simulink library "ChimeControlLibBtc"  (R2022b)
settings: Solver=VariableStepAuto  StartTime=0.0  StopTime=10.0  RelTol=1e-3
undefined symbols (not defined in the file or in its folder): chime_group_count, Row, spkrRouting
libraries: dspindex x10, RTC x3, FeaturePath x2, TOP x2, TuneVar x2, HandyTextFile x1
(part 1 of 2)
settings Model: Creator=kl13806  LastModifiedBy=kl13806
settings SolverCC: AlgebraicLoopSolver=TrustRegion
settings DebuggingCC: UnconnectedInputMsg=warning  UnconnectedOutputMsg=warning  UnconnectedLineMsg=warning  SFMachineParentedDataDiag=warning
settings ModelReferenceCC: EnableRefExpFcnMdlSchedulingChecks=on
settings RTWCC: DLArmComputeVersion=19.05

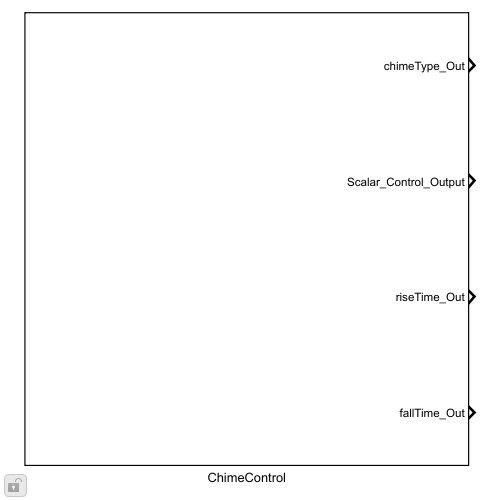
[thumbnail: Simulink's stored preview of the top-level diagram]
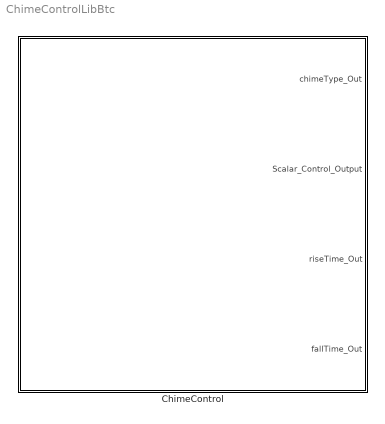
== system ChimeControlLibBtc ==
  ChimeControl : Subsystem  mask(Chimes ChimeControl){Config=[], FeatureName=Control}
      mask prompts: Config "ChimeControlConfig"; FeatureName "Feature path name:"
      mask init:
      | blkh=gcbh;
      | Config=BTConfig.Assert(blkh,Config);
      | 
      | Config.Validate();
      | BTConfig.InitSetFeatureIfPresent(blkh,'FeatureName');
      | 
      | % Flatten variables used by MFBs:
      | %nch=Config.Nch;
      mask Callback Config: BTConfig.CallbackHideIfPresent(gcbh,{'FeatureName'});
      mask TypeOptions FeatureName: FeaturePath/FeatureName

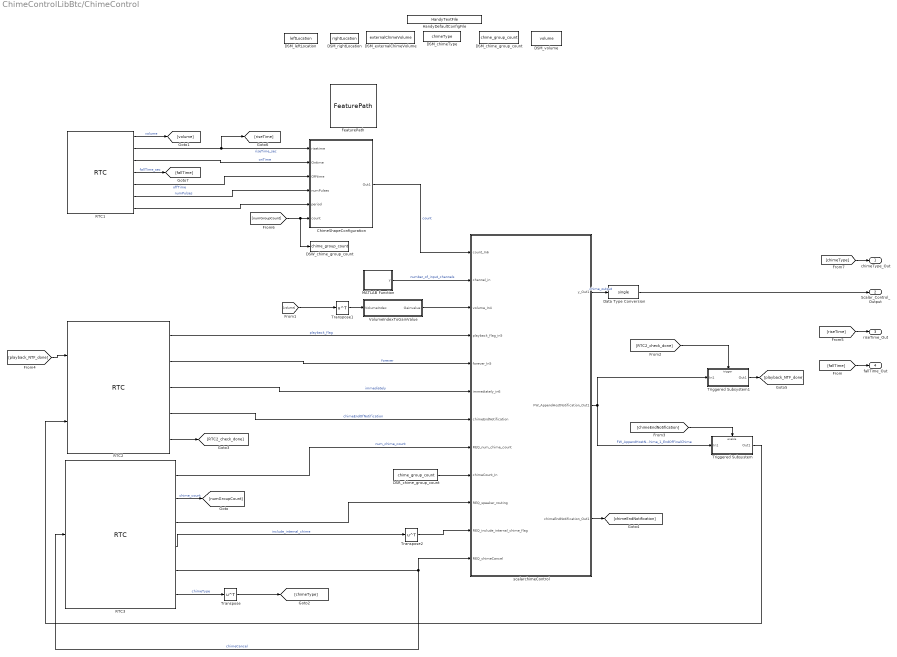
== system ChimeControlLibBtc/ChimeControl ==
  ChimeShapeConfiguration : Subsystem
  DSM_chimeType : DataStoreMemory  DataStoreName=chimeType  ShowAdditionalParam=off
  DSM_chime_group_count : DataStoreMemory  DataStoreName=chime_group_count  InitialValue=ones(1, Config.Nch)  ShowAdditionalParam=off
  DSM_externalChimeVolume : DataStoreMemory  DataStoreName=externalChimeVolume  InitialValue=zeros(1,Config.Nch)  ShowAdditionalParam=off
  DSM_leftLocation : DataStoreMemory  DataStoreName=leftLocation  ShowAdditionalParam=off
  DSM_rightLocation : DataStoreMemory  DataStoreName=rightLocation  ShowAdditionalParam=off
  DSM_volume : DataStoreMemory  DataStoreName=volume  InitialValue=Config.Volume  ShowAdditionalParam=off
  DSR_chime_group_count : DataStoreRead  DataStoreName=chime_group_count  IndexOptions=Index vector (dialog)  Indices=1  OutputSizes=1
  DSW_chime_group_count : DataStoreWrite  DataStoreName=chime_group_count  IndexOptions=Index vector (dialog)  Indices=1  OutputSizes=1
  Data Type Conversion : DataTypeConversion  OutDataTypeStr=single  SaturateOnIntegerOverflow=off  RndMeth=Floor
  FeaturePath : FeaturePath/FeaturePath  FeatureName=Control  IsGroup=off  GroupNumber=-1  IsModule=off  TriggerInit=[800 149 915 256]
  HandyDefaultConfigFile : HandyTextFile/HandyTextFile  TemplateSource=Config  FileSuffix=Init  OpenDialogOnLoad=off  UseThisBlockName=off  TheDefaultText=|  ShowInLibBrowser=on
      | % $(FILENAME) Setup model parameters for each "Init" callback (e.g. update diagram)
      | sample_rate_in_hertz = 44100;
      | frame_size = 32;
      | sysin_channel_count = 2;
  MATLAB Function : MATLAB Function  TreatAsAtomicUnit=on
  RTC1 : RTC/RTC  REQ_Priority=RTC_Mask.NormalPriority  RequestAtInit=off  EnableRequest=off  REQElemName1=volume  REQElemType1=single  REQElemWidth1=length(Config.Volume)  REQElemInitial1=Config.Volume  REQElemName2=riseTime  REQElemType2=single  REQElemWidth2=length(Config.RiseTime)  REQElemInitial2=Config.RiseTime  REQElemName3=onTime  REQElemType3=single  REQElemWidth3=length(Config.OnTime)  REQElemInitial3=Config.OnTime  REQElemName4=fallTime  REQElemType4=single  REQElemWidth4=length(Config.FallTime)  REQElemInitial4=Config.FallTime  REQElemName5=offTime  REQElemType5=single  REQElemWidth5=length(Config.OffTime)  REQElemInitial5=Config.OffTime  REQElemName6=numPulses  REQElemType6=int32  REQElemWidth6=length(Config.NumPulses)  REQElemInitial6=Config.NumPulses  REQElemName7=period  REQElemType7=single  REQElemWidth7=length(Config.Period)  REQElemInitial7=Config.Period  REQElemType8=uint32  REQElemWidth8=1  REQElemInitial8=[]  REQElemType9=uint32  REQElemWidth9=1  REQElemInitial9=[]  REQElemType10=uint32  REQElemWidth10=1  REQElemInitial10=[]  EnableResponse=on  EnableRSP_StatusIn=off  RSPElemType1=uint32  RSPElemWidth1=1  RSPElemType2=uint32  RSPElemWidth2=1  RSPElemType3=uint32  RSPElemWidth3=1  RSPElemType4=uint32  RSPElemWidth4=1  RSPElemType5=uint32  RSPElemWidth5=1  RSPElemType6=uint32  RSPElemWidth6=1  RSPElemType7=uint32  RSPElemWidth7=1  RSPElemType8=uint32  RSPElemWidth8=1  RSPElemType9=uint32  RSPElemWidth9=1  RSPElemType10=uint32  RSPElemWidth10=1  EnableNotification=off  EnableNTF_PrepTrig=off  NTFElemType1=uint32  NTFElemWidth1=1  NTFElemType2=uint32  NTFElemWidth2=1  NTFElemType3=uint32  NTFElemWidth3=1  NTFElemType4=uint32  NTFElemWidth4=1  NTFElemType5=uint32  NTFElemWidth5=1  NTFElemType6=uint32  NTFElemWidth6=1  NTFElemType7=uint32  NTFElemWidth7=1  NTFElemType8=uint32  NTFElemWidth8=1  NTFElemType9=uint32  NTFElemWidth9=1  NTFElemType10=uint32  NTFElemWidth10=1  MaskMessageName=PulseConfig
  RTC2 : RTC/RTC  REQ_Priority=RTC_Mask.NormalPriority  RequestAtInit=off  EnableRequest=off  REQElemName1=PlaybackSignal  REQElemType1=int32  REQElemWidth1=length(Config.PlaybackFlag)  REQElemInitial1=Config.PlaybackFlag  REQElemName2=Forever  REQElemType2=boolean  REQElemWidth2=length(Config.Forever)  REQElemInitial2=Config.Forever  REQElemName3=Immediately  REQElemType3=boolean  REQElemWidth3=length(Config.Immediately)  REQElemInitial3=Config.Immediately  REQElemName4=ChimeEndNotification  REQElemType4=boolean  REQElemWidth4=length(Config.ChimeEndNotification)  REQElemInitial4=Config.ChimeEndNotification  REQElemType5=uint32  REQElemWidth5=1  REQElemInitial5=[]  REQElemType6=uint32  REQElemWidth6=1  REQElemInitial6=[]  REQElemType7=uint32  REQElemWidth7=1  REQElemInitial7=[]  REQElemType8=uint32  REQElemWidth8=1  REQElemInitial8=[]  REQElemType9=uint32  REQElemWidth9=1  REQElemInitial9=[]  REQElemType10=uint32  REQElemWidth10=1  REQElemInitial10=[]  EnableResponse=on  EnableRSP_StatusIn=off  RSPElemType1=uint32  RSPElemWidth1=1  RSPElemType2=uint32  RSPElemWidth2=1  RSPElemType3=uint32  RSPElemWidth3=1  RSPElemType4=uint32  RSPElemWidth4=1  RSPElemType5=uint32  RSPElemWidth5=1  RSPElemType6=uint32  RSPElemWidth6=1  RSPElemType7=uint32  RSPElemWidth7=1  RSPElemType8=uint32  RSPElemWidth8=1  RSPElemType9=uint32  RSPElemWidth9=1  RSPElemType10=uint32  RSPElemWidth10=1  EnableNotification=on  EnableNTF_PrepTrig=off  NTFElemName1=FW_AppendHostNotification  NTFElemType1=boolean  NTFElemWidth1=length(Config.ChimeEndNotification)  NTFElemType2=uint32  NTFElemWidth2=1  NTFElemType3=uint32  NTFElemWidth3=1  NTFElemType4=uint32  NTFElemWidth4=1  NTFElemType5=uint32  NTFElemWidth5=1  NTFElemType6=uint32  NTFElemWidth6=1  NTFElemType7=uint32  NTFElemWidth7=1  NTFElemType8=uint32  NTFElemWidth8=1  NTFElemType9=uint32  NTFElemWidth9=1  NTFElemType10=uint32  NTFElemWidth10=1  MaskMessageName=StatePlayback
  RTC3 : RTC/RTC  REQ_Priority=RTC_Mask.NormalPriority  RequestAtInit=off  EnableRequest=off  REQElemName1=NumChimeCount  REQElemType1=int32  REQElemWidth1=length(Config.NumChimeCount)  REQElemInitial1=Config.NumChimeCount  REQElemName2=NumGroupCount  REQElemType2=int32  REQElemWidth2=length(chime_group_count)  REQElemInitial2=chime_group_count  REQElemName3=SpeakerRouting  REQElemType3=int32  REQElemWidth3=length(spkrRouting)  REQElemInitial3=spkrRouting  REQElemName4=IncludeInternalChimeFlag  REQElemType4=boolean  REQElemWidth4=length(Config.IncludeInternalChimeFlag)  REQElemInitial4=Config.IncludeInternalChimeFlag  REQElemName5=ChimeCancel  REQElemType5=boolean  REQElemWidth5=length(Config.ChimeCancel)  REQElemInitial5=Config.ChimeCancel  REQElemName6=ChimeType  REQElemType6=single  REQElemWidth6=length(Config.ChimeType)  REQElemInitial6=Config.ChimeType  REQElemType7=boolean  REQElemWidth7=1  REQElemInitial7=[]  REQElemType8=int32  REQElemWidth8=1  REQElemInitial8=[]  REQElemType9=int32  REQElemWidth9=1  REQElemInitial9=[]  REQElemType10=int32  REQElemWidth10=1  REQElemInitial10=[]  EnableResponse=on  EnableRSP_StatusIn=off  RSPElemName1=chimeCancelAck  RSPElemType1=boolean  RSPElemWidth1=length(Config.ChimeCancel)  RSPElemType2=uint32  RSPElemWidth2=1  RSPElemType3=uint32  RSPElemWidth3=1  RSPElemType4=uint32  RSPElemWidth4=1  RSPElemType5=uint32  RSPElemWidth5=1  RSPElemType6=uint32  RSPElemWidth6=1  RSPElemType7=uint32  RSPElemWidth7=1  RSPElemType8=uint32  RSPElemWidth8=1  RSPElemType9=uint32  RSPElemWidth9=1  RSPElemType10=uint32  RSPElemWidth10=1  EnableNotification=off  EnableNTF_PrepTrig=off  NTFElemType1=uint32  NTFElemWidth1=1  NTFElemType2=uint32  NTFElemWidth2=1  NTFElemType3=uint32  NTFElemWidth3=1  NTFElemType4=uint32  NTFElemWidth4=1  NTFElemType5=uint32  NTFElemWidth5=1  NTFElemType6=uint32  NTFElemWidth6=1  NTFElemType7=uint32  NTFElemWidth7=1  NTFElemType8=uint32  NTFElemWidth8=1  NTFElemType9=uint32  NTFElemWidth9=1  NTFElemType10=uint32  NTFElemWidth10=1  MaskMessageName=ChimesFeature
  Transpose : Math  Operator=transpose  SignedPower=on
  Transpose1 : Math  Operator=transpose  SignedPower=on
  Transpose2 : Math  Operator=transpose  SignedPower=on
  Triggered Subsystem : Subsystem  TreatAsAtomicUnit=on
  Triggered Subsystem1 : Subsystem  TreatAsAtomicUnit=on
  VolumeIndexToGainValue : Subsystem
  scalarchimeControl : Subsystem
  chimeType_Out : Outport  VectorParamsAs1DForOutWhenUnconnected=off
  Scalar_Control_Output : Outport  Port=2  VectorParamsAs1DForOutWhenUnconnected=off
  riseTime_Out : Outport  Port=3  VectorParamsAs1DForOutWhenUnconnected=off
  fallTime_Out : Outport  Port=4  VectorParamsAs1DForOutWhenUnconnected=off
  wires:
  Data Type Conversion/1 -> Scalar_Control_Output/1
  VolumeIndexToGainValue/1(Gainvalue) -> scalarchimeControl/3(volume_In4)
  RTC1/2 -> ChimeShapeConfiguration/1(risetime), [riseTime]  "riseTime_sec"
  RTC2/3 -> scalarchimeControl/6(immediately_in6)  "immediately"
  RTC3/5 -> scalarchimeControl/12(REQ_chimeCancel), RTC3/1  "chimeCancel"
  scalarchimeControl/1(y_Out1) -> Data Type Conversion/1  "chime_output"
  RTC2/1 -> scalarchimeControl/4(playback_flag_in5)  "playback_flag"
  Transpose2/1 -> scalarchimeControl/11(REQ_include_internal_chime_flag)
  RTC1/3 -> ChimeShapeConfiguration/2(Ontime)  "onTime"
  DSR_chime_group_count/1 -> scalarchimeControl/9(chimeCount_In)
  RTC3/1 -> scalarchimeControl/8(REQ_num_chime_count)  "num_chime_count"
  RTC2/4 -> scalarchimeControl/7(chimeEndNotification)  "chimeEndOfNotification"
  ChimeShapeConfiguration/1(Out1) -> scalarchimeControl/1(count_In6)  "count"
  RTC2/2 -> scalarchimeControl/5(forever_In5)  "forever"
  Transpose1/1 -> VolumeIndexToGainValue/1(VolumeIndex)
  Triggered Subsystem/1(Out1) -> RTC2/2
  RTC1/5 -> ChimeShapeConfiguration/3(Offtime)  "offTime"
  RTC3/6 -> Transpose/1  "chimeType"
  scalarchimeControl/2(FW_AppendHostNotification_Out1) -> Triggered Subsystem/1(In1), Triggered Subsystem1/1(In1)  "FW_AppendHostNotification_0_StartOfFinalChime_1_EndOfFinalChime"
  RTC3/4 -> Transpose2/1  "include_internal_chime"
  RTC3/3 -> scalarchimeControl/10(REQ_speaker_routing)
  RTC1/7 -> ChimeShapeConfiguration/5(period)
  RTC1/1 -> [volume]  "volume"
  [volume] -> Transpose1/1
  Transpose/1 -> [chimeType]
  RTC2/5 -> [RTC2_check_done]
  [RTC2_check_done] -> Triggered Subsystem1/Trigger
  scalarchimeControl/3(chimeEndNotification_Out1) -> [chimeEndNotification]
  [chimeEndNotification] -> Triggered Subsystem/Enable
  Triggered Subsystem1/1(Out1) -> [playback_NTF_done]
  [playback_NTF_done] -> RTC2/1
  RTC1/6 -> ChimeShapeConfiguration/4(numPulses)  "numPulses"
  RTC1/4 -> [fallTime]  "fallTime_sec"
  [riseTime] -> riseTime_Out/1
  [fallTime] -> fallTime_Out/1
  RTC3/2 -> [numGroupCount]  "chime_count"
  [numGroupCount] -> DSW_chime_group_count/1, ChimeShapeConfiguration/6(count)
  [chimeType] -> chimeType_Out/1
  MATLAB Function/1(y) -> scalarchimeControl/2(channel_in)  "number_of_input_channels"

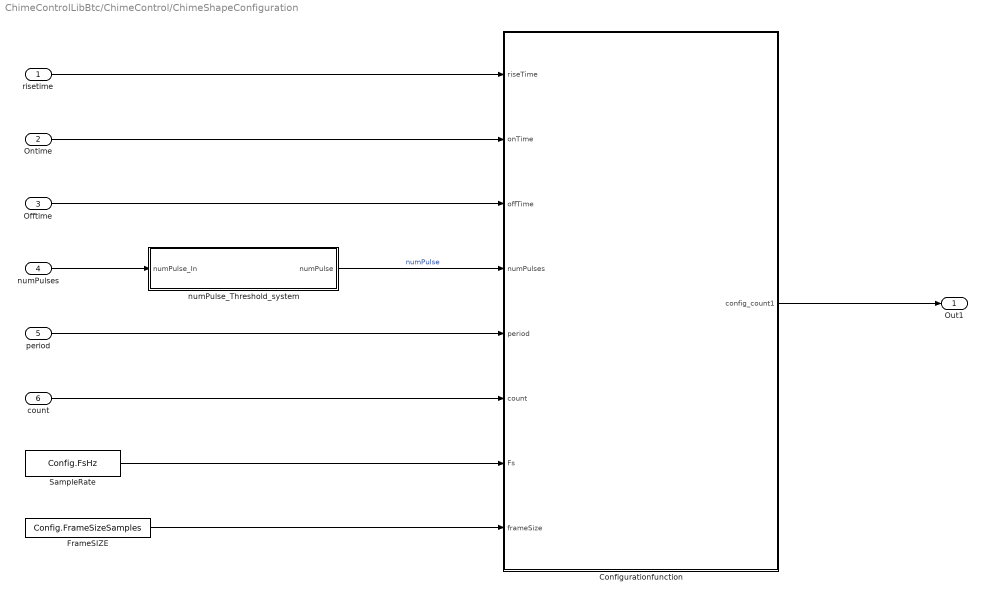
== system ChimeControlLibBtc/ChimeControl/ChimeShapeConfiguration ==
  risetime : Inport
  Ontime : Inport  Port=2
  Offtime : Inport  Port=3
  numPulses : Inport  Port=4
  period : Inport  Port=5
  count : Inport  Port=6
  Configurationfunction : MATLAB Function  TreatAsAtomicUnit=on
  FrameSIZE : Constant  Value=Config.FrameSizeSamples  OutDataTypeStr=single
  SampleRate : Constant  Value=Config.FsHz  OutDataTypeStr=single
  numPulse_Threshold_system : Subsystem
  Out1 : Outport  VectorParamsAs1DForOutWhenUnconnected=off
  wires:
  FrameSIZE/1 -> Configurationfunction/8(frameSize)
  SampleRate/1 -> Configurationfunction/7(Fs)
  count/1 -> Configurationfunction/6(count)
  Offtime/1 -> Configurationfunction/3(offTime)
  Configurationfunction/1(config_count1) -> Out1/1
  period/1 -> Configurationfunction/5(period)
  Ontime/1 -> Configurationfunction/2(onTime)
  risetime/1 -> Configurationfunction/1(riseTime)
  numPulses/1 -> numPulse_Threshold_system/1(numPulse_In)
  numPulse_Threshold_system/1(numPulse) -> Configurationfunction/4(numPulses)  "numPulse"

== system ChimeControlLibBtc/ChimeControl/Triggered Subsystem ==
  In1 : Inport
  Enable : EnablePort
  Data Type Conversion : DataTypeConversion  OutDataTypeStr=int32  SaturateOnIntegerOverflow=off  RndMeth=Floor
  Out1 : Outport  VectorParamsAs1DForOutWhenUnconnected=off
  wires:
  In1/1 -> Data Type Conversion/1
  Data Type Conversion/1 -> Out1/1

== system ChimeControlLibBtc/ChimeControl/Triggered Subsystem1 ==
  In1 : Inport
  Trigger : TriggerPort  TriggerType=function-call  VariantControl=Variant
  Constant : Constant
  Equal : RelationalOperator  Operator===  OutDataTypeStr=boolean  RndMeth=Simplest  InputSameDT=off
  Variable Selector : dspindex/Variable Selector  NumInputs=1  rowsOrCols=Columns  IdxMode=Fixed  Elements=[1]  ZerOneIdxMode=One-based  errmode=Clip Index  FillMode=on  FillValues=0
  Out1 : Outport  VectorParamsAs1DForOutWhenUnconnected=off
  wires:
  Variable Selector/1 -> Out1/1
  Constant/1 -> Equal/2
  Equal/1 -> Variable Selector/1
  In1/1 -> Equal/1

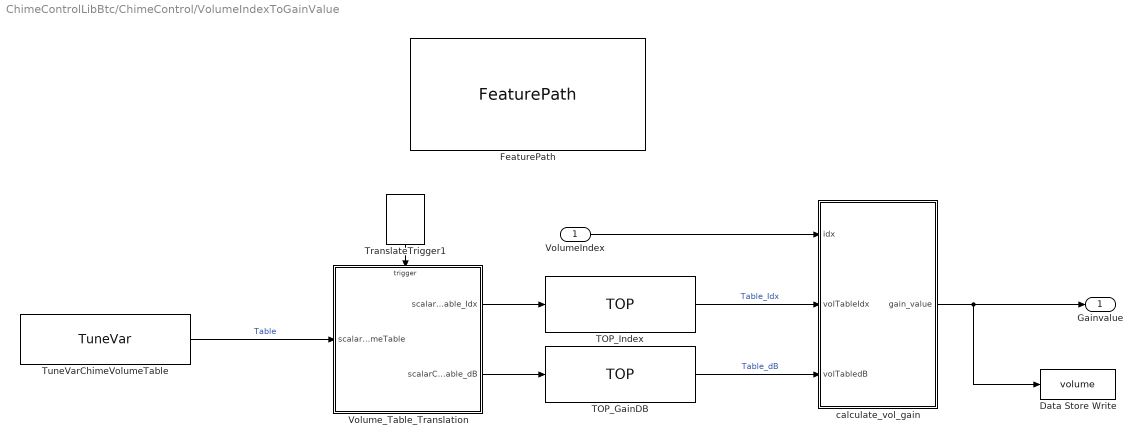
== system ChimeControlLibBtc/ChimeControl/VolumeIndexToGainValue ==
  VolumeIndex : Inport
  Data Store Write : DataStoreWrite  DataStoreName=volume  IndexOptions=Index vector (dialog)  Indices=1  OutputSizes=1
  FeaturePath : FeaturePath/FeaturePath  FeatureName=chimeVolume  IsGroup=off  GroupNumber=-1  IsModule=off  TriggerInit=[360 -1 595 111]
  TOP_GainDB : TOP/TOP  TriggerInit=[495 307 645 363]  TopName=Table_dB  DataType=Inherit: Same as input  BankNumber=0  PreOverlay=false  PostOverlay=false  Role=Automatic
  TOP_Index : TOP/TOP  TriggerInit=[495 237 645 293]  TopName=Table_Idx  DataType=Inherit: Same as input  BankNumber=0  PreOverlay=false  PostOverlay=false  Role=Automatic
  TranslateTrigger1 : TuneVar/TranslateTrigger  TriggerInit=[336 155 374 205]
  TuneVarChimeVolumeTable : TuneVar/TuneVar  Description=|  TuneName=Table  SpecifyMaxSize=off  VariableDim=1 (Row)  MaxSize=[2 11]  TunabilityNumber=2  MinValue=[0;-100]  MaxValue=[1;0]  TriggerInit=[-30 275 140 325]  MaskValue=[[1 32 64 96 128 160 192 224 230 240 250] / 255; [-126.5 -100 -90 -40 -30 -20 -10 0.0 6.0206 10 20]]
      | <HTML>Gain table maps index to gain.
      | The index values are <FONT color="red">normalized</Font> floats between 0 and 1 while the gains are in dB (i.e. 0 implies no attenuation).
      | </html>
  Volume_Table_Translation : MATLAB Function  TreatAsAtomicUnit=on
  calculate_vol_gain : MATLAB Function  TreatAsAtomicUnit=on
  Gainvalue : Outport  VectorParamsAs1DForOutWhenUnconnected=off
  wires:
  TOP_GainDB/1 -> calculate_vol_gain/3(volTabledB)  "Table_dB"
  Volume_Table_Translation/2(scalarChimeControl_Table_dB) -> TOP_GainDB/1
  TuneVarChimeVolumeTable/1 -> Volume_Table_Translation/1(scalarChimeControl_VolumeTable)  "Table"
  Volume_Table_Translation/1(scalarChimeControl_Table_Idx) -> TOP_Index/1
  TOP_Index/1 -> calculate_vol_gain/2(volTableIdx)  "Table_Idx"
  calculate_vol_gain/1(gain_value) -> Data Store Write/1, Gainvalue/1
  TranslateTrigger1/1 -> Volume_Table_Translation/Trigger
  VolumeIndex/1 -> calculate_vol_gain/1(idx)

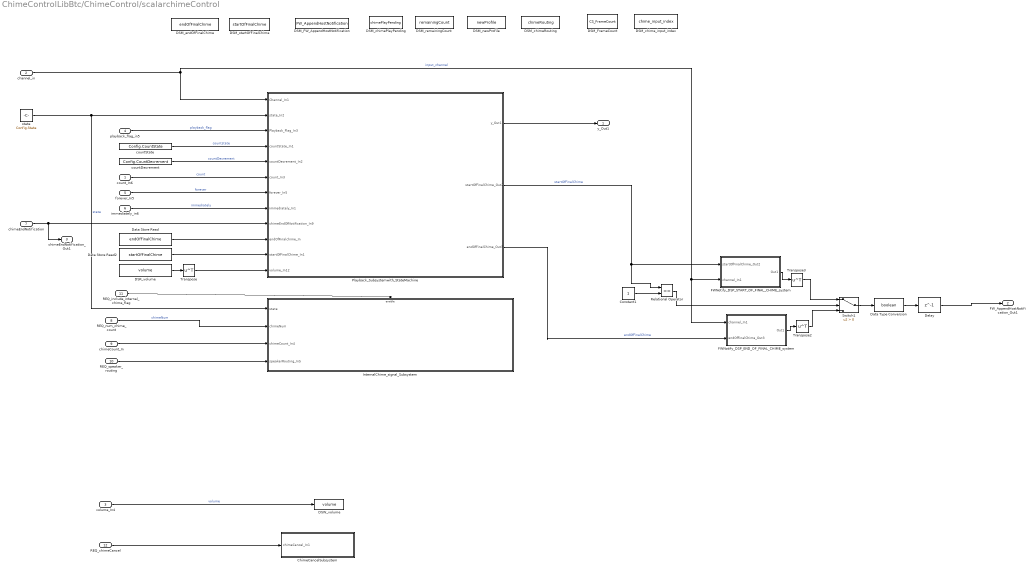
== system ChimeControlLibBtc/ChimeControl/scalarchimeControl ==
  count_In6 : Inport
  channel_in : Inport  Port=2
  volume_In4 : Inport  Port=3
  playback_flag_in5 : Inport  Port=4
  forever_In5 : Inport  Port=5
  immediately_in6 : Inport  Port=6
  chimeEndNotification : Inport  Port=7
  REQ_num_chime_count : Inport  Port=8
  chimeCount_In : Inport  Port=9
  REQ_speaker_routing : Inport  Port=10
  REQ_include_internal_chime_flag : Inport  Port=11
  REQ_chimeCancel : Inport  Port=12
  ChimeCancelSubsystem : Subsystem
  Constant1 : Constant  OutDataTypeStr=single
  DSM_FW_AppendHostNotification : DataStoreMemory  DataStoreName=FW_AppendHostNotification  InitialValue=zeros(1,Config.Nch)  ShowAdditionalParam=off
  DSM_FrameCount : DataStoreMemory  DataStoreName=CS_FrameCount  ShowAdditionalParam=off  OutDataTypeStr=int32
  DSM_chimePlayPending : DataStoreMemory  DataStoreName=chimePlayPending  InitialValue=zeros(1,Config.Nch)  ShowAdditionalParam=off  OutDataTypeStr=int32
  DSM_chimeRouting : DataStoreMemory  DataStoreName=chimeRouting  InitialValue=zeros(1,Config.Nch)  ShowAdditionalParam=off  OutDataTypeStr=int32
  DSM_chime_input_index : DataStoreMemory  DataStoreName=chime_input_index  InitialValue=Config.ChimeInputIndex  ShowAdditionalParam=off
  DSM_endOfFinalChime : DataStoreMemory  DataStoreName=endOfFinalChime  InitialValue=zeros(1,Config.Nch)  VectorParams1D=off  ShowAdditionalParam=off  OutDataTypeStr=boolean
  DSM_newProfile : DataStoreMemory  DataStoreName=newProfile  ShowAdditionalParam=off  OutDataTypeStr=int32
  DSM_remainingCount : DataStoreMemory  DataStoreName=remainingCount  ShowAdditionalParam=off  OutDataTypeStr=int32
  DSM_startOfFinalChime : DataStoreMemory  DataStoreName=startOfFinalChime  InitialValue=zeros(1,Config.Nch)  VectorParams1D=off  ShowAdditionalParam=off  OutDataTypeStr=boolean
  DSR_volume : DataStoreRead  DataStoreName=volume  IndexOptions=Index vector (dialog)  Indices=1  OutputSizes=1
  DSW_volume : DataStoreWrite  DataStoreName=volume  IndexOptions=Index vector (dialog)  Indices=1  OutputSizes=1
  Data Store Read : DataStoreRead  DataStoreName=endOfFinalChime  IndexOptions=Index vector (dialog)  Indices=1  OutputSizes=1
  Data Store Read2 : DataStoreRead  DataStoreName=startOfFinalChime  IndexOptions=Index vector (dialog)  Indices=1  OutputSizes=1
  Data Type Conversion : DataTypeConversion  OutDataTypeStr=boolean  SaturateOnIntegerOverflow=off  RndMeth=Floor
  Delay : Delay  DelayLength=1  InputProcessing=Columns as channels (frame based)
  FWNotify_DSP_END_OF_FINAL_CHIME_system : Subsystem  TreatAsAtomicUnit=on
  FWNotify_DSP_START_OF_FINAL_CHIME_system : Subsystem  TreatAsAtomicUnit=on
  InternalChime_signal_Subsystem : Subsystem
  Playback_Subsystemwith_StateMachine : Subsystem
  Relational Operator : RelationalOperator  Operator===  OutDataTypeStr=boolean  RndMeth=Simplest  InputSameDT=off
  Switch1 : Switch  Criteria=u2 > Threshold  SaturateOnIntegerOverflow=off  InputSameDT=off
  Transpose : Math  Operator=transpose  SignedPower=on
  Transpose2 : Math  Operator=transpose  SignedPower=on
  Transpose3 : Math  Operator=transpose  SignedPower=on
  countDecrement : Constant  Value=Config.CountDecrement  VectorParams1D=off  OutDataTypeStr=single
  countState : Constant  Value=Config.CountState  VectorParams1D=off  OutDataTypeStr=single
  state : Constant  Value=Config.State  VectorParams1D=off  OutDataTypeStr=single
  y_Out1 : Outport  VectorParamsAs1DForOutWhenUnconnected=off
  FW_AppendHostNotification_Out1 : Outport  Port=2  VectorParamsAs1DForOutWhenUnconnected=off
  chimeEndNotification_Out1 : Outport  Port=3  VectorParamsAs1DForOutWhenUnconnected=off
  wires:
  Constant1/1 -> Relational Operator/2
  Data Store Read2/1 -> Playback_Subsystemwith_StateMachine/11(startOfFinalChime_In1)
  Transpose/1 -> Playback_Subsystemwith_StateMachine/12(volume_In12)
  DSR_volume/1 -> Transpose/1
  volume_In4/1 -> DSW_volume/1  "volume"
  Data Store Read/1 -> Playback_Subsystemwith_StateMachine/10(endOfFinalchime_In)
  REQ_speaker_routing/1 -> InternalChime_signal_Subsystem/4(speakerRouting_In5)
  chimeCount_In/1 -> InternalChime_signal_Subsystem/3(chimeCount_In4)
  Playback_Subsystemwith_StateMachine/2(startOfFinalChime_Out2) -> Relational Operator/1, FWNotify_DSP_START_OF_FINAL_CHIME_system/1(startOfFinalChime_Out2)  "startOfFinalChime"
  Playback_Subsystemwith_StateMachine/3(endOfFinalChime_Out3) -> FWNotify_DSP_END_OF_FINAL_CHIME_system/2(endOfFinalChime_Out3)  "endOfFinalChime"
  chimeEndNotification/1 -> chimeEndNotification_Out1/1, Playback_Subsystemwith_StateMachine/9(chimeEndOfNotification_In9)
  countState/1 -> Playback_Subsystemwith_StateMachine/4(countState_In1)  "countstate"
  immediately_in6/1 -> Playback_Subsystemwith_StateMachine/8(immediately_In1)  "immediately"
  forever_In5/1 -> Playback_Subsystemwith_StateMachine/7(forever_In5)  "forever"
  count_In6/1 -> Playback_Subsystemwith_StateMachine/6(count_In3)  "count"
  countDecrement/1 -> Playback_Subsystemwith_StateMachine/5(countDecrement_In2)  "countDecrement"
  playback_flag_in5/1 -> Playback_Subsystemwith_StateMachine/3(Playback_Flag_In3)  "playback_flag"
  state/1 -> Playback_Subsystemwith_StateMachine/2(state_In2), InternalChime_signal_Subsystem/1(state)  "state"
  Playback_Subsystemwith_StateMachine/1(y_Out1) -> y_Out1/1
  REQ_include_internal_chime_flag/1 -> InternalChime_signal_Subsystem/Enable
  REQ_num_chime_count/1 -> InternalChime_signal_Subsystem/2(chimeNum)  "chimeNum"
  REQ_chimeCancel/1 -> ChimeCancelSubsystem/1(chimeCancel_In1)
  FWNotify_DSP_START_OF_FINAL_CHIME_system/1(Out1) -> Transpose3/1
  Transpose3/1 -> Switch1/1
  Delay/1 -> FW_AppendHostNotification_Out1/1
  channel_in/1 -> FWNotify_DSP_END_OF_FINAL_CHIME_system/1(channel_In1), FWNotify_DSP_START_OF_FINAL_CHIME_system/2(channel_In1), Playback_Subsystemwith_StateMachine/1(Channel_In1)  "input_channel"
  Switch1/1 -> Data Type Conversion/1
  FWNotify_DSP_END_OF_FINAL_CHIME_system/1(Out1) -> Transpose2/1
  Transpose2/1 -> Switch1/3
  Data Type Conversion/1 -> Delay/1
  Relational Operator/1 -> Switch1/2

== system ChimeControlLibBtc/ChimeControl/ChimeShapeConfiguration/numPulse_Threshold_system ==
  numPulse_In : Inport
  If Action Subsystem : Subsystem  TreatAsAtomicUnit=on
  If Action Subsystem1 : Subsystem  TreatAsAtomicUnit=on
  Relational Operator : RelationalOperator  OutDataTypeStr=boolean  RndMeth=Simplest  InputSameDT=off
  Switch : Switch  Criteria=u2 ~= 0  SaturateOnIntegerOverflow=off  InputSameDT=off
  thresholdNumPulse : Constant  Value=Config.ThresholdNumPulse  VectorParams1D=off  OutDataTypeStr=single
  numPulse : Outport  VectorParamsAs1DForOutWhenUnconnected=off
  wires:
  If Action Subsystem1/1(Out1) -> Switch/3
  If Action Subsystem/1(Out1) -> Switch/1
  Relational Operator/1 -> Switch/2
  Switch/1 -> numPulse/1  "numPulse"
  numPulse_In/1 -> If Action Subsystem/1(In1), Relational Operator/1
  thresholdNumPulse/1 -> If Action Subsystem1/1(In1), Relational Operator/2

== system ChimeControlLibBtc/ChimeControl/scalarchimeControl/ChimeCancelSubsystem ==
  chimeCancel_In1 : Inport
  If : If  IfExpression=u1 == 1
  If Action Subsystem : Subsystem  TreatAsAtomicUnit=on
  If Action Subsystem1 : Subsystem  TreatAsAtomicUnit=on
  wires:
  chimeCancel_In1/1 -> If/1
  If/1 -> If Action Subsystem/Action
  If/2 -> If Action Subsystem1/Action

== system ChimeControlLibBtc/ChimeControl/scalarchimeControl/FWNotify_DSP_END_OF_FINAL_CHIME_system ==
  channel_In1 : Inport
  endOfFinalChime_Out3 : Inport  Port=2
  Assignment : Assignment  DiagnosticForDimensions=Warning  IndexOptions=Index vector (port)  Indices=1  OutputSizes=1
  Assignment1 : Assignment  DiagnosticForDimensions=Warning  IndexOptions=Index vector (port)  Indices=1  OutputSizes=1
  Constant : Constant  VectorParams1D=off  OutDataTypeStr=single
  DSR_FW_AppendHostNotification : DataStoreRead  DataStoreName=FW_AppendHostNotification  IndexOptions=Index vector (dialog)  Indices=1  OutputSizes=1
  DSW_endOfFinalChime : DataStoreWrite  DataStoreName=endOfFinalChime  IndexOptions=Index vector (dialog)  Indices=1  OutputSizes=1
  Data Type Conversion : DataTypeConversion  OutDataTypeStr=boolean  SaturateOnIntegerOverflow=off  RndMeth=Floor
  Out1 : Outport  VectorParamsAs1DForOutWhenUnconnected=off
  wires:
  channel_In1/1 -> Assignment1/3, Assignment/3
  DSR_FW_AppendHostNotification/1 -> Assignment/1
  Constant/1 -> Data Type Conversion/1, Assignment/2
  Assignment/1 -> Out1/1
  Data Type Conversion/1 -> Assignment1/2
  Assignment1/1 -> DSW_endOfFinalChime/1
  endOfFinalChime_Out3/1 -> Assignment1/1

== system ChimeControlLibBtc/ChimeControl/scalarchimeControl/FWNotify_DSP_START_OF_FINAL_CHIME_system ==
  startOfFinalChime_Out2 : Inport
  channel_In1 : Inport  Port=2
  Assignment : Assignment  DiagnosticForDimensions=Warning  IndexOptions=Index vector (port)  Indices=1  OutputSizes=1
  Assignment1 : Assignment  DiagnosticForDimensions=Warning  IndexOptions=Index vector (port)  Indices=1  OutputSizes=1
  Constant : Constant  Value=0  OutDataTypeStr=single
  DSR_FW_AppendHostNotification : DataStoreRead  DataStoreName=FW_AppendHostNotification  IndexOptions=Index vector (dialog)  Indices=1  OutputSizes=1
  Data Store Write : DataStoreWrite  DataStoreName=startOfFinalChime  IndexOptions=Index vector (dialog)  Indices=1  OutputSizes=1
  Data Type Conversion : DataTypeConversion  OutDataTypeStr=boolean  SaturateOnIntegerOverflow=off  RndMeth=Floor
  Out1 : Outport  VectorParamsAs1DForOutWhenUnconnected=off
  wires:
  channel_In1/1 -> Assignment1/3, Assignment/3
  DSR_FW_AppendHostNotification/1 -> Assignment/1
  Constant/1 -> Data Type Conversion/1, Assignment/2
  Assignment/1 -> Out1/1
  Data Type Conversion/1 -> Assignment1/2
  Assignment1/1 -> Data Store Write/1
  startOfFinalChime_Out2/1 -> Assignment1/1

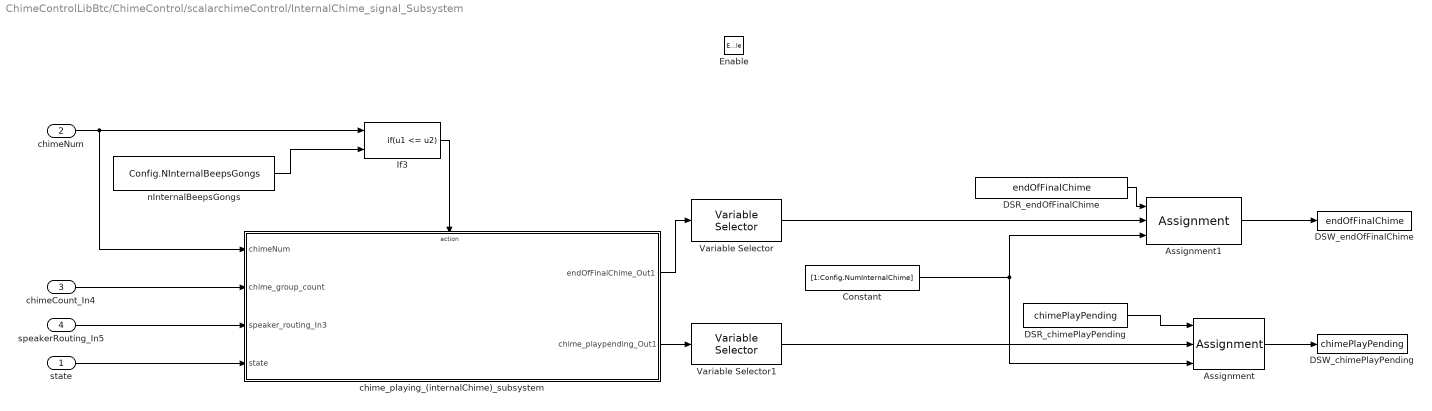
== system ChimeControlLibBtc/ChimeControl/scalarchimeControl/InternalChime_signal_Subsystem ==
  state : Inport
  chimeNum : Inport  Port=2
  chimeCount_In4 : Inport  Port=3
  speakerRouting_In5 : Inport  Port=4
  Enable : EnablePort
  Assignment : Assignment  DiagnosticForDimensions=Warning  IndexOptions=Index vector (port)  Indices=1  OutputSizes=1
  Assignment1 : Assignment  DiagnosticForDimensions=Warning  IndexOptions=Index vector (port)  Indices=1  OutputSizes=1
  Constant : Constant  Value=[1:Config.NumInternalChime]  OutDataTypeStr=single
  DSR_chimePlayPending : DataStoreRead  DataStoreName=chimePlayPending  IndexOptions=Index vector (dialog)  Indices=1  OutputSizes=1
  DSR_endOfFinalChime : DataStoreRead  DataStoreName=endOfFinalChime  IndexOptions=Index vector (dialog)  Indices=1  OutputSizes=1
  DSW_chimePlayPending : DataStoreWrite  DataStoreName=chimePlayPending  IndexOptions=Index vector (dialog)  Indices=1  OutputSizes=1
  DSW_endOfFinalChime : DataStoreWrite  DataStoreName=endOfFinalChime  IndexOptions=Index vector (dialog)  Indices=1  OutputSizes=1
  If3 : If  NumInputs=2  IfExpression=u1 <= u2  ShowElse=off
  Variable Selector : dspindex/Variable Selector  NumInputs=1  rowsOrCols=Columns  IdxMode=Fixed  Elements=[1:Config.NumInternalChime]  ZerOneIdxMode=One-based  errmode=Clip Index  FillMode=on  FillValues=0
  Variable Selector1 : dspindex/Variable Selector  NumInputs=1  rowsOrCols=Columns  IdxMode=Fixed  Elements=[1:Config.NumInternalChime]  ZerOneIdxMode=One-based  errmode=Clip Index  FillMode=on  FillValues=0
  chime_playing_(internalChime)_subsystem : Subsystem
  nInternalBeepsGongs : Constant  Value=Config.NInternalBeepsGongs  OutDataTypeStr=int32
  wires:
  If3/1 -> chime_playing_(internalChime)_subsystem/Action
  chimeCount_In4/1 -> chime_playing_(internalChime)_subsystem/2(chime_group_count)
  state/1 -> chime_playing_(internalChime)_subsystem/4(state)
  nInternalBeepsGongs/1 -> If3/2
  speakerRouting_In5/1 -> chime_playing_(internalChime)_subsystem/3(speaker_routing_In3)
  chimeNum/1 -> chime_playing_(internalChime)_subsystem/1(chimeNum), If3/1
  chime_playing_(internalChime)_subsystem/1(endOfFinalChime_Out1) -> Variable Selector/1
  chime_playing_(internalChime)_subsystem/2(chime_playpending_Out1) -> Variable Selector1/1
  Variable Selector/1 -> Assignment1/2
  Assignment1/1 -> DSW_endOfFinalChime/1
  Assignment/1 -> DSW_chimePlayPending/1
  DSR_chimePlayPending/1 -> Assignment/1
  Variable Selector1/1 -> Assignment/2
  DSR_endOfFinalChime/1 -> Assignment1/1
  Constant/1 -> Assignment/3, Assignment1/3

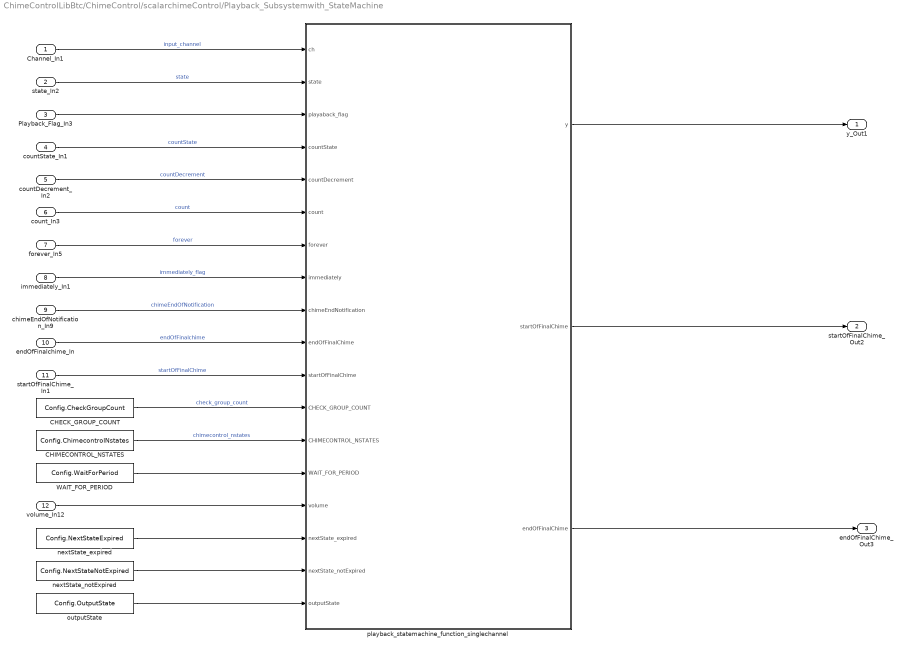
== system ChimeControlLibBtc/ChimeControl/scalarchimeControl/Playback_Subsystemwith_StateMachine ==
  Channel_In1 : Inport
  state_In2 : Inport  Port=2
  Playback_Flag_In3 : Inport  Port=3
  countState_In1 : Inport  Port=4
  countDecrement_In2 : Inport  Port=5
  count_In3 : Inport  Port=6
  forever_In5 : Inport  Port=7
  immediately_In1 : Inport  Port=8
  chimeEndOfNotification_In9 : Inport  Port=9
  endOfFinalchime_In : Inport  Port=10
  startOfFinalChime_In1 : Inport  Port=11
  volume_In12 : Inport  Port=12
  CHECK_GROUP_COUNT : Constant  Value=Config.CheckGroupCount  VectorParams1D=off  OutDataTypeStr=single
  CHIMECONTROL_NSTATES : Constant  Value=Config.ChimecontrolNstates  VectorParams1D=off  OutDataTypeStr=single
  WAIT_FOR_PERIOD : Constant  Value=Config.WaitForPeriod  VectorParams1D=off  OutDataTypeStr=single
  nextState_expired : Constant  Value=Config.NextStateExpired  OutDataTypeStr=single
  nextState_notExpired : Constant  Value=Config.NextStateNotExpired  OutDataTypeStr=single
  outputState : Constant  Value=Config.OutputState  OutDataTypeStr=single
  playback_statemachine_function_singlechannel : MATLAB Function  TreatAsAtomicUnit=on
  y_Out1 : Outport  VectorParamsAs1DForOutWhenUnconnected=off
  startOfFinalChime_Out2 : Outport  Port=2  VectorParamsAs1DForOutWhenUnconnected=off
  endOfFinalChime_Out3 : Outport  Port=3  VectorParamsAs1DForOutWhenUnconnected=off
  wires:
  count_In3/1 -> playback_statemachine_function_singlechannel/6(count)  "count"
  volume_In12/1 -> playback_statemachine_function_singlechannel/15(volume)
  nextState_notExpired/1 -> playback_statemachine_function_singlechannel/17(nextState_notExpired)
  nextState_expired/1 -> playback_statemachine_function_singlechannel/16(nextState_expired)
  outputState/1 -> playback_statemachine_function_singlechannel/18(outputState)
  WAIT_FOR_PERIOD/1 -> playback_statemachine_function_singlechannel/14(WAIT_FOR_PERIOD)
  playback_statemachine_function_singlechannel/1(y) -> y_Out1/1
  playback_statemachine_function_singlechannel/2(startOfFinalChime) -> startOfFinalChime_Out2/1
  playback_statemachine_function_singlechannel/3(endOfFinalChime) -> endOfFinalChime_Out3/1
  Channel_In1/1 -> playback_statemachine_function_singlechannel/1(ch)  "input_channel"
  CHECK_GROUP_COUNT/1 -> playback_statemachine_function_singlechannel/12(CHECK_GROUP_COUNT)  "check_group_count"
  CHIMECONTROL_NSTATES/1 -> playback_statemachine_function_singlechannel/13(CHIMECONTROL_NSTATES)  "chimecontrol_nstates"
  startOfFinalChime_In1/1 -> playback_statemachine_function_singlechannel/11("startOfFinalChime ")  "startOfFinalChime"
  countDecrement_In2/1 -> playback_statemachine_function_singlechannel/5(countDecrement)  "countDecrement"
  chimeEndOfNotification_In9/1 -> playback_statemachine_function_singlechannel/9(chimeEndNotification)  "chimeEndOfNotification"
  immediately_In1/1 -> playback_statemachine_function_singlechannel/8(immediately)  "immediately_flag"
  forever_In5/1 -> playback_statemachine_function_singlechannel/7(forever)  "forever"
  endOfFinalchime_In/1 -> playback_statemachine_function_singlechannel/10("endOfFinalChime ")  "endOfFinalchime"
  state_In2/1 -> playback_statemachine_function_singlechannel/2(state)  "state"
  Playback_Flag_In3/1 -> playback_statemachine_function_singlechannel/3(playaback_flag)
  countState_In1/1 -> playback_statemachine_function_singlechannel/4(countState)  "countState"

== system ChimeControlLibBtc/ChimeControl/ChimeShapeConfiguration/numPulse_Threshold_system/If Action Subsystem ==
  In1 : Inport
  Out1 : Outport  VectorParamsAs1DForOutWhenUnconnected=off
  wires:
  In1/1 -> Out1/1

== system ChimeControlLibBtc/ChimeControl/ChimeShapeConfiguration/numPulse_Threshold_system/If Action Subsystem1 ==
  In1 : Inport
  Out1 : Outport  VectorParamsAs1DForOutWhenUnconnected=off
  wires:
  In1/1 -> Out1/1

== system ChimeControlLibBtc/ChimeControl/scalarchimeControl/ChimeCancelSubsystem/If Action Subsystem ==
  Action Port : ActionPort
  Assignment : Assignment  DiagnosticForDimensions=Warning  IndexOptions=Assign all  Indices=1  OutputSizes=1
  DSR_volume : DataStoreRead  DataStoreName=volume  IndexOptions=Index vector (dialog)  Indices=1  OutputSizes=1
  DSW_volume : DataStoreWrite  DataStoreName=volume  IndexOptions=Index vector (dialog)  Indices=1  OutputSizes=1
  MATLAB Function : MATLAB Function  TreatAsAtomicUnit=on
  wires:
  Assignment/1 -> DSW_volume/1
  DSR_volume/1 -> Assignment/1
  MATLAB Function/1(y) -> Assignment/2

== system ChimeControlLibBtc/ChimeControl/scalarchimeControl/ChimeCancelSubsystem/If Action Subsystem1 ==
  Action Port : ActionPort
  DSR_volume : DataStoreRead  DataStoreName=volume  IndexOptions=Index vector (dialog)  Indices=1  OutputSizes=1
  DSW_volume : DataStoreWrite  DataStoreName=volume  IndexOptions=Index vector (dialog)  Indices=1  OutputSizes=1
  wires:
  DSR_volume/1 -> DSW_volume/1

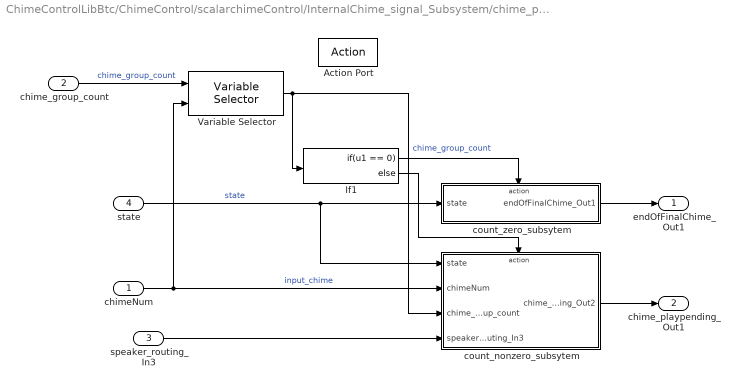
== system ChimeControlLibBtc/ChimeControl/scalarchimeControl/InternalChime_signal_Subsystem/chime_playing_(internalChime)_subsystem ==
  chimeNum : Inport
  chime_group_count : Inport  Port=2
  speaker_routing_In3 : Inport  Port=3
  state : Inport  Port=4
  Action Port : ActionPort
  If1 : If  IfExpression=u1 == 0
  Variable Selector : dspindex/Variable Selector  NumInputs=1  rowsOrCols=Columns  IdxMode=Variable  Elements=[1 3]  ZerOneIdxMode=One-based  errmode=Clip Index  FillMode=on  FillValues=0
  count_nonzero_subsytem : Subsystem  TreatAsAtomicUnit=on
  count_zero_subsytem : Subsystem  TreatAsAtomicUnit=on
  endOfFinalChime_Out1 : Outport  VectorParamsAs1DForOutWhenUnconnected=off
  chime_playpending_Out1 : Outport  Port=2  VectorParamsAs1DForOutWhenUnconnected=off
  wires:
  Variable Selector/1 -> If1/1, count_nonzero_subsytem/3(chime_group_count)  "chime_group_count"
  If1/1 -> count_zero_subsytem/Action
  state/1 -> count_nonzero_subsytem/1(state), count_zero_subsytem/1(state)  "state"
  chimeNum/1 -> Variable Selector/2, count_nonzero_subsytem/2(chimeNum)  "input_chime"
  speaker_routing_In3/1 -> count_nonzero_subsytem/4(speaker_routing_In3)
  If1/2 -> count_nonzero_subsytem/Action
  chime_group_count/1 -> Variable Selector/1  "chime_group_count"
  count_zero_subsytem/1(endOfFinalChime_Out1) -> endOfFinalChime_Out1/1
  count_nonzero_subsytem/1(chime_playpending_Out2) -> chime_playpending_Out1/1

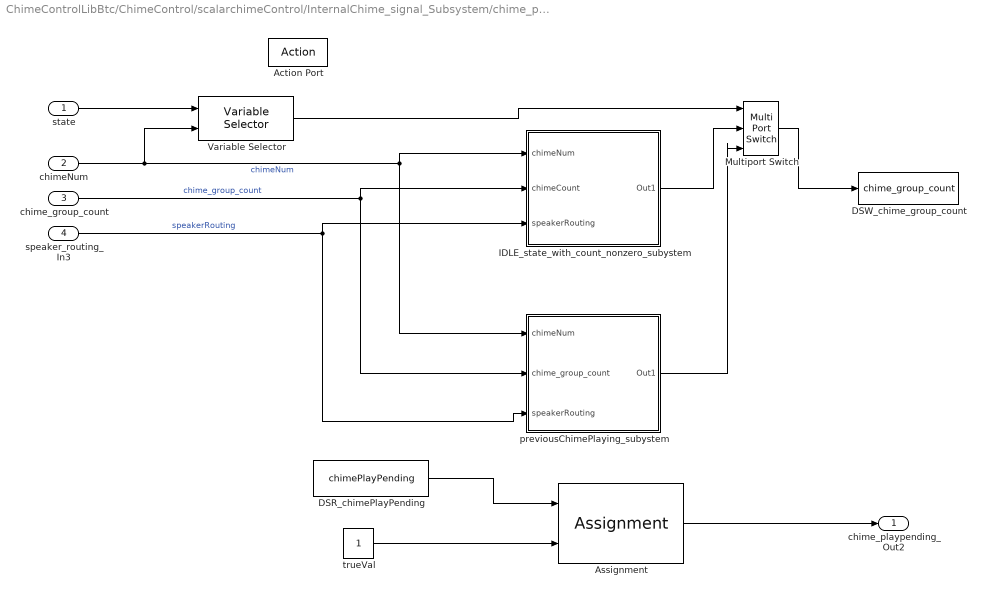
== system ChimeControlLibBtc/ChimeControl/scalarchimeControl/InternalChime_signal_Subsystem/chime_playing_(internalChime)_subsystem/count_nonzero_subsytem ==
  state : Inport
  chimeNum : Inport  Port=2
  chime_group_count : Inport  Port=3
  speaker_routing_In3 : Inport  Port=4
  Action Port : ActionPort
  Assignment : Assignment  DiagnosticForDimensions=Warning  IndexOptions=Assign all  Indices=1  OutputSizes=1
  DSR_chimePlayPending : DataStoreRead  DataStoreName=chimePlayPending  IndexOptions=Index vector (dialog)  Indices=1  OutputSizes=1
  DSW_chime_group_count : DataStoreWrite  DataStoreName=chime_group_count  IndexOptions=Index vector (dialog)  Indices=1  OutputSizes=1
  IDLE_state_with_count_nonzero_subystem : Subsystem  TreatAsAtomicUnit=on
  Multiport Switch : MultiPortSwitch  DataPortOrder=Zero-based contiguous  Inputs=2  zeroidx=on  SaturateOnIntegerOverflow=off  InputSameDT=off
  Variable Selector : dspindex/Variable Selector  NumInputs=1  rowsOrCols=Columns  IdxMode=Variable  Elements=[1 3]  ZerOneIdxMode=One-based  errmode=Clip Index  FillMode=on  FillValues=0
  previousChimePlaying_subystem : Subsystem  TreatAsAtomicUnit=on
  trueVal : Constant  OutDataTypeStr=int32
  chime_playpending_Out2 : Outport  VectorParamsAs1DForOutWhenUnconnected=off
  wires:
  state/1 -> Variable Selector/1
  chimeNum/1 -> Variable Selector/2, previousChimePlaying_subystem/1(chimeNum), IDLE_state_with_count_nonzero_subystem/1(chimeNum)  "chimeNum"
  chime_group_count/1 -> previousChimePlaying_subystem/2(chime_group_count), IDLE_state_with_count_nonzero_subystem/2(chimeCount)  "chime_group_count"
  speaker_routing_In3/1 -> previousChimePlaying_subystem/3(speakerRouting), IDLE_state_with_count_nonzero_subystem/3(speakerRouting)  "speakerRouting"
  DSR_chimePlayPending/1 -> Assignment/1
  trueVal/1 -> Assignment/2
  Assignment/1 -> chime_playpending_Out2/1
  IDLE_state_with_count_nonzero_subystem/1(Out1) -> Multiport Switch/2
  previousChimePlaying_subystem/1(Out1) -> Multiport Switch/3
  Multiport Switch/1 -> DSW_chime_group_count/1
  Variable Selector/1 -> Multiport Switch/1

== system ChimeControlLibBtc/ChimeControl/scalarchimeControl/InternalChime_signal_Subsystem/chime_playing_(internalChime)_subsystem/count_zero_subsytem ==
  state : Inport
  Action Port : ActionPort
  Multiport Switch : MultiPortSwitch  DataPortOrder=Zero-based contiguous  Inputs=2  zeroidx=on  SaturateOnIntegerOverflow=off  InputSameDT=off
  trueVal : Constant  OutDataTypeStr=boolean
  endOfFinalChime_Out1 : Outport  VectorParamsAs1DForOutWhenUnconnected=off
  wires:
  state/1 -> Multiport Switch/1
  Multiport Switch/1 -> endOfFinalChime_Out1/1
  trueVal/1 -> Multiport Switch/3, Multiport Switch/2

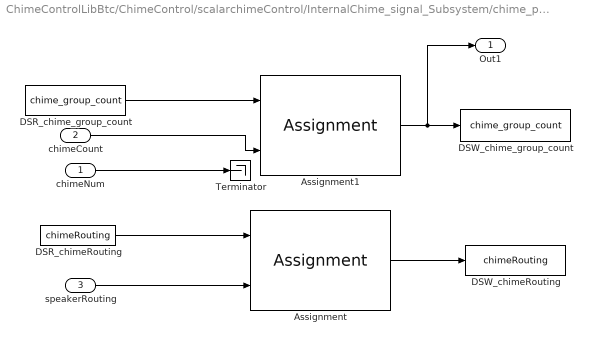
== system ChimeControlLibBtc/ChimeControl/scalarchimeControl/InternalChime_signal_Subsystem/chime_playing_(internalChime)_subsystem/count_nonzero_subsytem/IDLE_state_with_count_nonzero_subystem ==
  chimeNum : Inport
  chimeCount : Inport  Port=2
  speakerRouting : Inport  Port=3
  Assignment : Assignment  DiagnosticForDimensions=Warning  IndexOptions=Assign all  Indices=1  OutputSizes=1
  Assignment1 : Assignment  DiagnosticForDimensions=Warning  IndexOptions=Assign all  Indices=1  OutputSizes=1
  DSR_chimeRouting : DataStoreRead  DataStoreName=chimeRouting  IndexOptions=Index vector (dialog)  Indices=1  OutputSizes=1
  DSR_chime_group_count : DataStoreRead  DataStoreName=chime_group_count  IndexOptions=Index vector (dialog)  Indices=1  OutputSizes=1
  "DSW_chimeRouting " : DataStoreWrite  DataStoreName=chimeRouting  IndexOptions=Index vector (dialog)  Indices=1  OutputSizes=1
  DSW_chime_group_count : DataStoreWrite  DataStoreName=chime_group_count  IndexOptions=Index vector (dialog)  Indices=1  OutputSizes=1
  Terminator : Terminator
  Out1 : Outport  VectorParamsAs1DForOutWhenUnconnected=off
  wires:
  DSR_chimeRouting/1 -> Assignment/1
  chimeNum/1 -> Terminator/1
  speakerRouting/1 -> Assignment/2
  Assignment/1 -> "DSW_chimeRouting "/1
  chimeCount/1 -> Assignment1/2
  DSR_chime_group_count/1 -> Assignment1/1
  Assignment1/1 -> Out1/1, DSW_chime_group_count/1

== system ChimeControlLibBtc/ChimeControl/scalarchimeControl/InternalChime_signal_Subsystem/chime_playing_(internalChime)_subsystem/count_nonzero_subsytem/previousChimePlaying_subystem ==
  chimeNum : Inport
  chime_group_count : Inport  Port=2
  speakerRouting : Inport  Port=3
  Data Store Read : DataStoreRead  DataStoreName=newProfile  IndexOptions=Index vector (dialog)  Indices=1  OutputSizes=1
  If : If
  Merge : Merge
  Variable Selector : dspindex/Variable Selector  NumInputs=1  rowsOrCols=Columns  IdxMode=Variable  Elements=[1 3]  ZerOneIdxMode=One-based  errmode=Clip Index  FillMode=on  FillValues=0
  continuousPreviousChime_subsystem : Subsystem  TreatAsAtomicUnit=on
  supression_subsystem : Subsystem  TreatAsAtomicUnit=on
  Out1 : Outport  VectorParamsAs1DForOutWhenUnconnected=off
  wires:
  chimeNum/1 -> Variable Selector/2, supression_subsystem/1(chimeNum), continuousPreviousChime_subsystem/1(chimeNum)  "chimeNum"
  Data Store Read/1 -> supression_subsystem/4(newProfile), Variable Selector/1
  Variable Selector/1 -> If/1
  If/1 -> supression_subsystem/Action
  chime_group_count/1 -> continuousPreviousChime_subsystem/2(chime_group_count), supression_subsystem/2(chimeCount)  "chimeCount"
  speakerRouting/1 -> continuousPreviousChime_subsystem/3(speakerRouting), supression_subsystem/3(speakerRouting)  "speakerRouting"
  If/2 -> continuousPreviousChime_subsystem/Action
  supression_subsystem/1(Out1) -> Merge/1
  continuousPreviousChime_subsystem/1(chimegroupCountOut1) -> Merge/2
  Merge/1 -> Out1/1

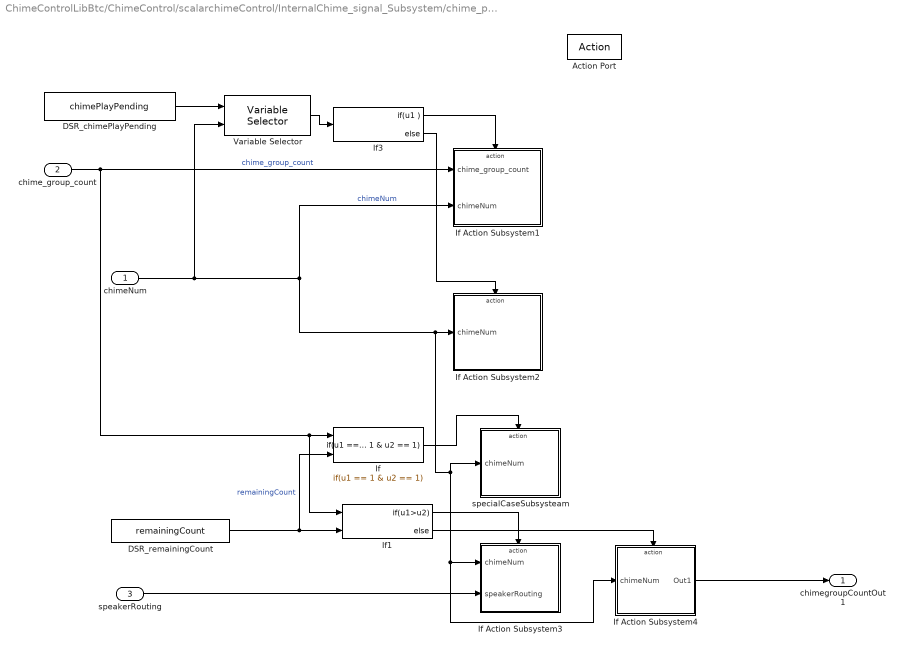
== system ChimeControlLibBtc/ChimeControl/scalarchimeControl/InternalChime_signal_Subsystem/chime_playing_(internalChime)_subsystem/count_nonzero_subsytem/previousChimePlaying_subystem/continuousPreviousChime_subsystem ==
  chimeNum : Inport
  chime_group_count : Inport  Port=2
  speakerRouting : Inport  Port=3
  Action Port : ActionPort
  DSR_chimePlayPending : DataStoreRead  DataStoreName=chimePlayPending  IndexOptions=Index vector (dialog)  Indices=1  OutputSizes=1
  DSR_remainingCount : DataStoreRead  DataStoreName=remainingCount  IndexOptions=Index vector (dialog)  Indices=1  OutputSizes=1
  If : If  NumInputs=2  IfExpression=u1 == 1 & u2 == 1  ShowElse=off
  If Action Subsystem1 : Subsystem  TreatAsAtomicUnit=on
  If Action Subsystem2 : Subsystem  TreatAsAtomicUnit=on
  If Action Subsystem3 : Subsystem  TreatAsAtomicUnit=on
  If Action Subsystem4 : Subsystem  TreatAsAtomicUnit=on
  If1 : If  NumInputs=2  IfExpression=u1>u2
  If3 : If  IfExpression=u1
  Variable Selector : dspindex/Variable Selector  NumInputs=1  rowsOrCols=Columns  IdxMode=Variable  Elements=[1 3]  ZerOneIdxMode=One-based  errmode=Clip Index  FillMode=on  FillValues=0
  specialCaseSubsysteam : Subsystem  TreatAsAtomicUnit=on
  chimegroupCountOut1 : Outport  VectorParamsAs1DForOutWhenUnconnected=off
  wires:
  If3/1 -> If Action Subsystem1/Action
  DSR_chimePlayPending/1 -> Variable Selector/1
  If3/2 -> If Action Subsystem2/Action
  chimeNum/1 -> Variable Selector/2, If Action Subsystem3/1(chimeNum), If Action Subsystem4/1(chimeNum), specialCaseSubsysteam/1(chimeNum), If Action Subsystem2/1(chimeNum), If Action Subsystem1/2(chimeNum)  "chimeNum"
  chime_group_count/1 -> If1/1, If/1, If Action Subsystem1/1(chime_group_count)  "chime_group_count"
  If/1 -> specialCaseSubsysteam/Action
  DSR_remainingCount/1 -> If/2, If1/2  "remainingCount"
  If1/1 -> If Action Subsystem3/Action
  speakerRouting/1 -> If Action Subsystem3/2(speakerRouting)
  If1/2 -> If Action Subsystem4/Action
  If Action Subsystem4/1(Out1) -> chimegroupCountOut1/1
  Variable Selector/1 -> If3/1

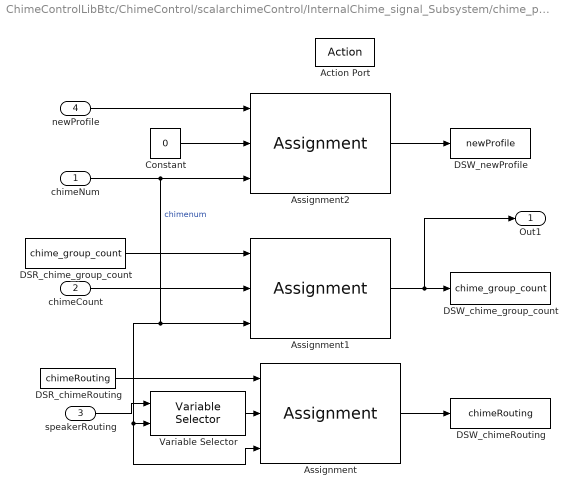
== system ChimeControlLibBtc/ChimeControl/scalarchimeControl/InternalChime_signal_Subsystem/chime_playing_(internalChime)_subsystem/count_nonzero_subsytem/previousChimePlaying_subystem/supression_subsystem ==
  chimeNum : Inport
  chimeCount : Inport  Port=2
  speakerRouting : Inport  Port=3
  newProfile : Inport  Port=4
  Action Port : ActionPort
  Assignment : Assignment  DiagnosticForDimensions=Warning  IndexOptions=Index vector (port)  Indices=1  OutputSizes=1
  Assignment1 : Assignment  DiagnosticForDimensions=Warning  IndexOptions=Index vector (port)  Indices=1  OutputSizes=1
  Assignment2 : Assignment  DiagnosticForDimensions=Warning  IndexOptions=Index vector (port)  Indices=1  OutputSizes=1
  Constant : Constant  Value=0  OutDataTypeStr=int32
  DSR_chimeRouting : DataStoreRead  DataStoreName=chimeRouting  IndexOptions=Index vector (dialog)  Indices=1  OutputSizes=1
  DSR_chime_group_count : DataStoreRead  DataStoreName=chime_group_count  IndexOptions=Index vector (dialog)  Indices=1  OutputSizes=1
  "DSW_chimeRouting " : DataStoreWrite  DataStoreName=chimeRouting  IndexOptions=Index vector (dialog)  Indices=1  OutputSizes=1
  DSW_chime_group_count : DataStoreWrite  DataStoreName=chime_group_count  IndexOptions=Index vector (dialog)  Indices=1  OutputSizes=1
  DSW_newProfile : DataStoreWrite  DataStoreName=newProfile  IndexOptions=Index vector (dialog)  Indices=1  OutputSizes=1
  Variable Selector : dspindex/Variable Selector  NumInputs=1  rowsOrCols=Columns  IdxMode=Variable  Elements=[1 3]  ZerOneIdxMode=One-based  errmode=Clip Index  FillMode=on  FillValues=0
  Out1 : Outport  VectorParamsAs1DForOutWhenUnconnected=off
  wires:
  DSR_chimeRouting/1 -> Assignment/1
  Assignment/1 -> "DSW_chimeRouting "/1
  Assignment1/1 -> DSW_chime_group_count/1, Out1/1
  chimeCount/1 -> Assignment1/2
  chimeNum/1 -> Assignment2/3, Assignment/3, Variable Selector/2, Assignment1/3  "chimenum"
  speakerRouting/1 -> Variable Selector/1
  DSR_chime_group_count/1 -> Assignment1/1
  newProfile/1 -> Assignment2/1
  Constant/1 -> Assignment2/2
  Assignment2/1 -> DSW_newProfile/1
  Variable Selector/1 -> Assignment/2

== system ChimeControlLibBtc/ChimeControl/scalarchimeControl/InternalChime_signal_Subsystem/chime_playing_(internalChime)_subsystem/count_nonzero_subsytem/previousChimePlaying_subystem/continuousPreviousChime_subsystem/If Action Subsystem1 ==
  chime_group_count : Inport
  chimeNum : Inport  Port=2
  Action Port : ActionPort
  DSW_remainingCount : DataStoreWrite  DataStoreName=remainingCount  IndexOptions=Index vector (dialog)  Indices=1  OutputSizes=1
  Variable Selector : dspindex/Variable Selector  NumInputs=1  rowsOrCols=Columns  IdxMode=Variable  Elements=[1 3]  ZerOneIdxMode=One-based  errmode=Clip Index  FillMode=on  FillValues=0
  wires:
  chime_group_count/1 -> Variable Selector/1
  chimeNum/1 -> Variable Selector/2  "chimeNum"
  Variable Selector/1 -> DSW_remainingCount/1

== system ChimeControlLibBtc/ChimeControl/scalarchimeControl/InternalChime_signal_Subsystem/chime_playing_(internalChime)_subsystem/count_nonzero_subsytem/previousChimePlaying_subystem/continuousPreviousChime_subsystem/If Action Subsystem2 ==
  chimeNum : Inport
  Action Port : ActionPort
  Add : Sum
  CHECK_GROUP_COUNT : Constant  Value=Config.CheckGroupCount  OutDataTypeStr=single
  CHIMECONTROL_NSTATES : Constant  Value=Config.ChimecontrolNstates  OutDataTypeStr=single
  DSW_remainingCount : DataStoreWrite  DataStoreName=remainingCount  IndexOptions=Index vector (dialog)  Indices=1  OutputSizes=1
  Data Type Conversion : DataTypeConversion  OutDataTypeStr=int32  SaturateOnIntegerOverflow=off  RndMeth=Floor
  Multiply : Product
  wires:
  Data Type Conversion/1 -> DSW_remainingCount/1
  chimeNum/1 -> Multiply/1
  CHIMECONTROL_NSTATES/1 -> Multiply/2
  Multiply/1 -> Add/1
  CHECK_GROUP_COUNT/1 -> Add/2
  Add/1 -> Data Type Conversion/1

== system ChimeControlLibBtc/ChimeControl/scalarchimeControl/InternalChime_signal_Subsystem/chime_playing_(internalChime)_subsystem/count_nonzero_subsytem/previousChimePlaying_subystem/continuousPreviousChime_subsystem/If Action Subsystem3 ==
  chimeNum : Inport
  speakerRouting : Inport  Port=2
  Action Port : ActionPort
  Assignment : Assignment  DiagnosticForDimensions=Warning  IndexOptions=Index vector (port)  Indices=1  OutputSizes=1
  DSR_chimeRouting : DataStoreRead  DataStoreName=chimeRouting  IndexOptions=Index vector (dialog)  Indices=1  OutputSizes=1
  DSW_chimeRouting : DataStoreWrite  DataStoreName=chimeRouting  IndexOptions=Index vector (dialog)  Indices=1  OutputSizes=1
  Variable Selector : dspindex/Variable Selector  NumInputs=1  rowsOrCols=Columns  IdxMode=Variable  Elements=[1 3]  ZerOneIdxMode=One-based  errmode=Clip Index  FillMode=on  FillValues=0
  wires:
  chimeNum/1 -> Variable Selector/2, Assignment/3
  DSR_chimeRouting/1 -> Assignment/1
  speakerRouting/1 -> Variable Selector/1
  Assignment/1 -> DSW_chimeRouting/1
  Variable Selector/1 -> Assignment/2

== system ChimeControlLibBtc/ChimeControl/scalarchimeControl/InternalChime_signal_Subsystem/chime_playing_(internalChime)_subsystem/count_nonzero_subsytem/previousChimePlaying_subystem/continuousPreviousChime_subsystem/If Action Subsystem4 ==
  chimeNum : Inport
  Action Port : ActionPort
  Assignment : Assignment  DiagnosticForDimensions=Warning  IndexOptions=Assign all  Indices=1  OutputSizes=1
  DSR_chime_group_count : DataStoreRead  DataStoreName=chime_group_count  IndexOptions=Index vector (dialog)  Indices=1  OutputSizes=1
  DSR_remainingCount : DataStoreRead  DataStoreName=remainingCount  IndexOptions=Index vector (dialog)  Indices=1  OutputSizes=1
  DSW_chime_group_count : DataStoreWrite  DataStoreName=chime_group_count  IndexOptions=Index vector (dialog)  Indices=1  OutputSizes=1
  Terminator : Terminator
  Out1 : Outport  VectorParamsAs1DForOutWhenUnconnected=off
  wires:
  chimeNum/1 -> Terminator/1
  DSR_chime_group_count/1 -> Assignment/1
  Assignment/1 -> Out1/1, DSW_chime_group_count/1
  DSR_remainingCount/1 -> Assignment/2

== system ChimeControlLibBtc/ChimeControl/scalarchimeControl/InternalChime_signal_Subsystem/chime_playing_(internalChime)_subsystem/count_nonzero_subsytem/previousChimePlaying_subystem/continuousPreviousChime_subsystem/specialCaseSubsysteam ==
  chimeNum : Inport
  Action Port : ActionPort
  Assignment : Assignment  DiagnosticForDimensions=Warning  IndexOptions=Index vector (port)  Indices=1  OutputSizes=1
  DSR_startOfFinalChime : DataStoreRead  DataStoreName=startOfFinalChime  IndexOptions=Index vector (dialog)  Indices=1  OutputSizes=1
  DSW_startOfFinalChime : DataStoreWrite  DataStoreName=startOfFinalChime  IndexOptions=Index vector (dialog)  Indices=1  OutputSizes=1
  trueVal : Constant  OutDataTypeStr=boolean
  wires:
  chimeNum/1 -> Assignment/3
  DSR_startOfFinalChime/1 -> Assignment/1
  trueVal/1 -> Assignment/2
  Assignment/1 -> DSW_startOfFinalChime/1
